simulink model "InversorPV_simple"  (R2017a)
settings: Solver=ode23  StartTime=0.0  StopTime=inf  MaxStep=1e-4  RelTol=1e-3
libraries: instrumentlib x1, powerlib x1
settings Model: Creator=MarioAndres  LastModifiedBy=AndrewB

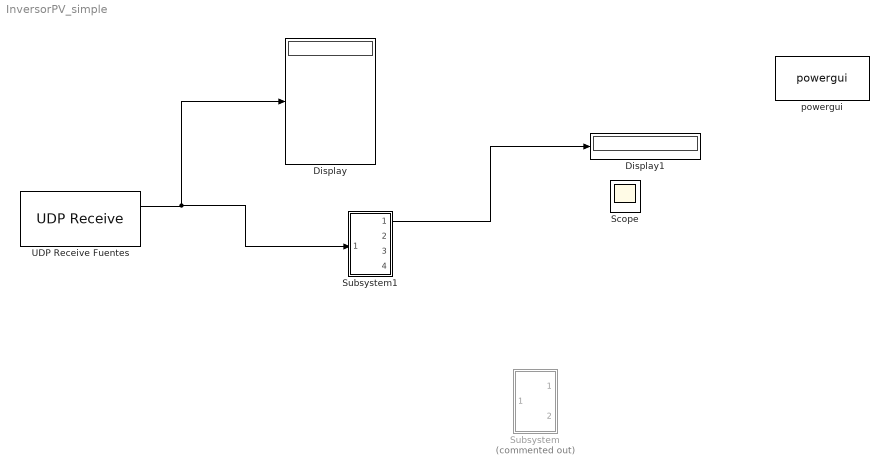
== system InversorPV_simple ==
  Display : Display
  Display1 : Display
  Scope : Scope
  Subsystem : Subsystem  Commented=on
  Subsystem1 : Subsystem
  UDP Receive Fuentes : instrumentlib/UDP Receive  Host=169.254.205.197  Port=51000  LocalPort=51001  DataSize="[6  1]"  EnableBlockingMode=off  Timeout=1  SampleTime=1  DataType=uint8  ByteOrder=BigEndian
      settings: SourceProductName=Instrument Control Toolbox
  powergui : powerlib/powergui  SimulationMode=Discrete  SampleTime=1/60/10000  frequency=60  Iterations=50  frequencyindice=0  Pbase=100e6  ErrMax=1e-4  UnitsV=kV  UnitsW=MW  buscounter=0  FunctionMessages=off  echomessages=off  EnableUseOfTLC=off  CurrentSourceSwitches=off  DisableSnubberDevices=off  DisableRonSwitches=off  DisableVfSwitches=off  DisplayEquations=off  SolverType=Tustin/Backward Euler (TBE)  Interpol=off  ExternalGateDelay=off  methode=off  Ts=100  x0status=blocks  SPID=on  SwTol=0  HookPort=off  RestoreLinks=warning  ResistiveCurrentMeasurement=off  Frange=[0:2:500]  Ylog=off  Xlog=on  ShowGrid=off  save=off  variable=ZData  structure=sps1phPWM1_str  ZoomFFT=on  StartTime=0.1-2/60  cycles=2  DisplayStyle=1  fundamental=60  FreqAxis=off  MaxFrequency=5000  frequencyindicesteady=1  RmsSteady=1  display=off
  wires:
  UDP Receive Fuentes/1 -> Subsystem1/1(In1), Display/1
  Subsystem1/1(Out1) -> Display1/1

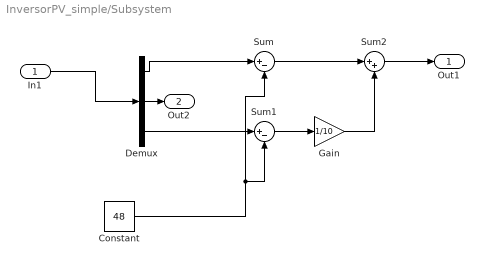
== system InversorPV_simple/Subsystem ==
  In1 : Inport
  Constant : Constant  Value=48
  Demux : Demux  Outputs=3
  Gain : Gain  Gain=1/10
  Sum : Sum  Inputs=|+-
  Sum1 : Sum  Inputs=|+-
  Sum2 : Sum  Inputs=|++
  Out1 : Outport
  Out2 : Outport  Port=2
  wires:
  Sum1/1 -> Gain/1
  Sum2/1 -> Out1/1
  Demux/1 -> Sum/1
  Gain/1 -> Sum2/2
  Constant/1 -> Sum/2, Sum1/2
  Sum/1 -> Sum2/1
  Demux/3 -> Sum1/1
  In1/1 -> Demux/1
  Demux/2 -> Out2/1

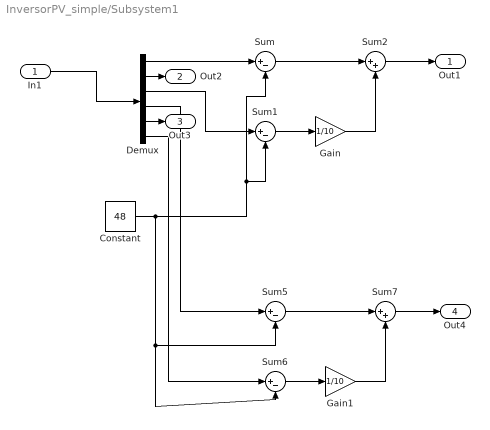
== system InversorPV_simple/Subsystem1 ==
  In1 : Inport
  Constant : Constant  Value=48
  Demux : Demux  Outputs=6
  Gain : Gain  Gain=1/10
  Gain1 : Gain  Gain=1/10
  Sum{,1,5..6} (4 alike) : Sum  Inputs=|+-
  Sum2 : Sum  Inputs=|++
  Sum7 : Sum  Inputs=|++
  Out1 : Outport
  Out2 : Outport  Port=2
  Out3 : Outport  Port=3
  Out4 : Outport  Port=4
  wires:
  Demux/1 -> Sum/1
  Gain/1 -> Sum2/2
  Sum2/1 -> Out1/1
  Sum6/1 -> Gain1/1
  Constant/1 -> Sum5/2, Sum6/2, Sum/2, Sum1/2
  Gain1/1 -> Sum7/2
  Demux/3 -> Sum1/1
  Sum5/1 -> Sum7/1
  Demux/6 -> Sum6/1
  Sum7/1 -> Out4/1
  Sum/1 -> Sum2/1
  Sum1/1 -> Gain/1
  Demux/4 -> Sum5/1
  Demux/5 -> Out3/1
  Demux/2 -> Out2/1
  In1/1 -> Demux/1
